simulink model "Sim_main"  (R2025a)
settings: Solver=FixedStepAuto  StartTime=0.0  StopTime=8760  FixedStep=1  RelTol=1e-3
values from neighbouring files (symbols this model uses):
  A = R * 2 * H    [LCOW_calculation.m]    (also in RUN_Simulink_POOL.m; RUN_Simulink_RandomSet.m; RUN_Simulink_SINGLE.m = 12.786871552)
  Cf = 36000    [RUN_Simulink_POOL.m]    (also in RUN_Simulink_RandomSet.m; RUN_Simulink_SINGLE.m)
  CutIn = 3    [RUN_Simulink_POOL.m]    (also in RUN_Simulink_RandomSet.m; RUN_Simulink_SINGLE.m)
  IP1 = (n/(n-1))*P1*( (P2/P1)^((n-1)/n) - 1)    (= 259255.992944)    [RUN_Simulink_POOL.m]    (also in RUN_Simulink_RandomSet.m; RUN_Simulink_SINGLE.m)
  J1 = 1.5 * As    [RUN_Simulink_POOL.m]    (also in RUN_Simulink_RandomSet.m; RUN_Simulink_SINGLE.m = 4.38)
  Limit_Tor = Tor_rq * 0.5    (= 2.3371585434)    [RUN_Simulink_POOL.m]    (also in RUN_Simulink_RandomSet.m; RUN_Simulink_SINGLE.m = 3.45899464424)
  N_PV = data.N_PV(i)    [LCOW_calculation.m]    (also in MOO_Qp_LCOW_CO2.m = optimvar("N_PV","Type","integer","LowerBound",1,"UpperBound"; RUN_Simulink_POOL.m = N_PV_values(i); RUN_Simulink_RandomSet.m = N_PV_values; RUN_Simulink_SINGLE.m = 2)
  N_ro = data.N_ro(i)    [LCOW_calculation.m]    (also in MOO_Qp_LCOW_CO2.m = optimvar("N_ro","Type","integer","LowerBound",2,"UpperBound"; RUN_Simulink_POOL.m = N_ro_values(i); RUN_Simulink_RandomSet.m = N_ro_values; RUN_Simulink_SINGLE.m = 6)
  Nt = data.Nt(i)    [LCOW_calculation.m]    (also in MOO_Qp_LCOW_CO2.m = optimvar("Nt","Type","integer","LowerBound",10,"UpperBound",; RUN_Simulink_POOL.m = Nt_values(i); RUN_Simulink_RandomSet.m = Nt_values; RUN_Simulink_SINGLE.m = 58)
  P2 = 800000    [RUN_Simulink_POOL.m]    (also in RUN_Simulink_RandomSet.m; RUN_Simulink_SINGLE.m)
  R = 0.515 * As    [LCOW_calculation.m]    (also in RUN_Simulink_POOL.m; RUN_Simulink_RandomSet.m; RUN_Simulink_SINGLE.m = 1.5038)
  Tor_rq = IP1 * Va * 10 / (17 * pi)    (= 4.67431708681)    [RUN_Simulink_POOL.m]    (also in RUN_Simulink_RandomSet.m; RUN_Simulink_SINGLE.m = 6.91798928848)
  TR = data.TR(i)    [LCOW_calculation.m]    (also in MOO_Qp_LCOW_CO2.m = optimvar("TR","LowerBound",3,"UpperBound",10); RUN_Simulink_POOL.m = TR_values(i); RUN_Simulink_RandomSet.m = TR_values; RUN_Simulink_SINGLE.m = 9.36)
  Va = e_vol * Vs    (= 9.6291546017e-05)    [RUN_Simulink_POOL.m]    (also in RUN_Simulink_RandomSet.m; RUN_Simulink_SINGLE.m = 0.000142511488105)
  Vf1 = ((P1+Pa)*T2/(T1*(P2+Pa)))*1000    (= 339.891157105)    [RUN_Simulink_POOL.m]    (also in RUN_Simulink_RandomSet.m; RUN_Simulink_SINGLE.m)
  Vt = 2000    [RUN_Simulink_POOL.m]    (also in RUN_Simulink_RandomSet.m; RUN_Simulink_SINGLE.m)
undefined symbols (not defined in the file or in its folder): magnitude
libraries: statsLibrary x36, simulink x1
(part 1 of 4)
settings Model: Creator=mep20kma  LastModifiedBy=mep20kma
settings DebuggingCC: AlgebraicLoopMsg=none

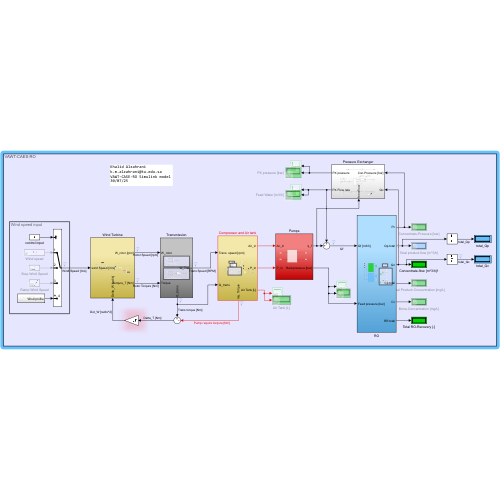
[thumbnail: Simulink's stored preview of the top-level diagram]
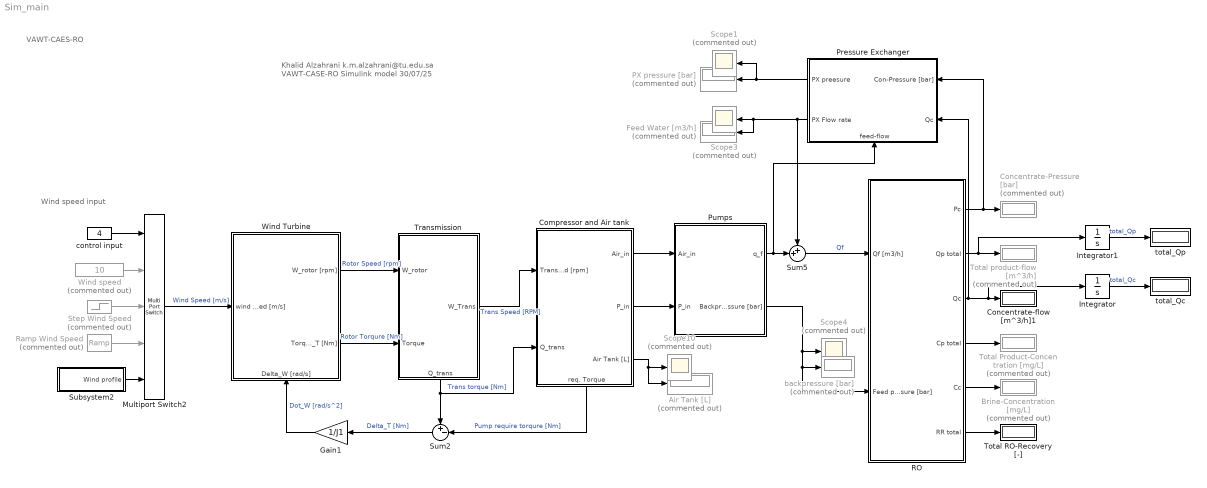
== system Sim_main ==
  note: Wind speed input
  note: VAWT-CAES-RO
  note: Khalid Alzahrani
      | k.m.alzahrani@tu.edu.sa
      | VAWT-CASE-RO Simulink model
      | 30/07/25
  Air Tank [L] : Display  Commented=on
      settings: Format=bank
  Brine-Concentration [mg/L] : Display  Commented=on
      settings: Format=bank
  Compressor and Air tank : Subsystem
      settings: PortSchema="{\"entries\":[{\"content\":{\"sides\":[{\"content\":{\"connectorIds\":[\"In1\",\"In2\"]},\"type\":\"ConnectorPlacement.EquallySpacedRectSide\",\"uuid\":\"bae99c5a-2a4b-4178-96fc-c8e23db237a2\"},{\"content\":{\"connectorIds\":[\"Out1\",\"Out2\",\"Out3\"],\"side\":\"RIGHT\"},\"type\":\"ConnectorPlacement.EquallySpacedRectSide\",\"uuid\":\"1992d0ba-6a8c-4d02-a787-c6c0cea2193f\"},{\"content\":{\"side\":\"TOP\"},\"type\":\"ConnectorPlacement.EquallySpacedRectSide\",\"uuid\":\"ca7b5cc6-18c4-4b8c-a524-0fed0e771665\"},{\"content\":{\"connectorIds\":[\"Out4\"],\"side\":\"BOTTOM\"},\"type\":\"ConnectorPlacement.EquallySpacedRectSide\",\"uuid\":\"cdfbee2c-ce1d-4f5d-a549-a4d701a0a4dd\"}]},\"type\":\"ConnectorPlacement.EquallySpacedConnector\",\"uuid\":\"eb75531c-d058-4587-8526-49bf71b34705\"}],\"packageUris\":[\"http://schema.mathworks.com/mf0/Connector/R2020b\"],\"version\":\"1.0\"}"
  Concentrate-Pressure [bar] : Display  Commented=on
  Concentrate-flow [m^3/h]1 : Display
      settings: Decimation=5
  Feed Water [m3/h] : Display  Commented=on
  Gain1 : Gain  Gain=1/J1
  Integrator : Integrator
  Integrator1 : Integrator  WrappedStateLowerValue=0.00000001
  Multiport Switch2 : MultiPortSwitch  Inputs=4  SaturateOnIntegerOverflow=off  InputSameDT=off
  PX pressure [bar] : Display  Commented=on
  Pressure Exchanger : Subsystem
      settings: PortSchema="{\"entries\":[{\"content\":{\"sides\":[{\"content\":{\"connectorIds\":[\"In1\",\"In2\"]},\"type\":\"ConnectorPlacement.EquallySpacedRectSide\",\"uuid\":\"0703a325-1e41-4562-9fad-9b159d1bd3be\"},{\"content\":{\"connectorIds\":[\"Out1\",\"Out2\"],\"side\":\"RIGHT\"},\"type\":\"ConnectorPlacement.EquallySpacedRectSide\",\"uuid\":\"c9b3212b-5369-47ef-bfa4-c3d90c4a3111\"},{\"content\":{\"side\":\"TOP\"},\"type\":\"ConnectorPlacement.EquallySpacedRectSide\",\"uuid\":\"f46ca4f0-02ad-4144-bb6a-e2761afa5cc2\"},{\"content\":{\"connectorIds\":[\"In3\"],\"side\":\"BOTTOM\"},\"type\":\"ConnectorPlacement.EquallySpacedRectSide\",\"uuid\":\"8b21c39f-2c5b-40be-94c0-35b7ce64feea\"}]},\"type\":\"ConnectorPlacement.EquallySpacedConnector\",\"uuid\":\"0ccfaa06-0329-44cf-a82f-b9aa7c53a6a3\"}],\"packageUris\":[\"http://schema.mathworks.com/mf0/Connector/R2020b\"],\"version\":\"1.0\"}"
  Pumps : Subsystem
  RO : Subsystem
  Ramp Wind Speed : simulink/Sources/Ramp  Commented=on  slope=0.1  start=0  InitialOutput=0
  Scope{1,3..4,10} (4 alike) : Scope  Commented=on
      Scope1 settings: ActiveDisplayYMinimum=-0.26427  ActiveDisplayYMaximum=2.37839  DataLoggingVariableName=ScopeData19
      Scope10 settings: ActiveDisplayYMinimum=-1627.2921760391182  ActiveDisplayYMaximum=23795.4869600652  DataLoggingVariableName=ScopeData22
      Scope3 settings: ActiveDisplayYMinimum=-6.500066936368408  ActiveDisplayYMaximum=58.500602427315691  DataLoggingVariableName=ScopeData32
      Scope4 settings: ActiveDisplayYMinimum=40.740007263636365  ActiveDisplayYMaximum=60.740007263636365  DataLoggingVariableName=ScopeData34
  Step Wind Speed : Step  Commented=on  After=6  SampleTime=1
  Subsystem2 : Subsystem
  Sum2 : Sum  Inputs=+-|
  Sum5 : Sum  Inputs=++|
  Total Product-Concentration [mg/L] : Display  Commented=on
  Total RO-Recovery [-] : Display
  Total product-flow [m^3/h] : Display  Commented=on
  Transmission : Subsystem
      settings: PortSchema="{\"entries\":[{\"content\":{\"sides\":[{\"content\":{\"connectorIds\":[\"In1\",\"In2\"]},\"type\":\"ConnectorPlacement.EquallySpacedRectSide\",\"uuid\":\"fe7cb8fe-c3d1-4fc2-abbc-e62d8a30f932\"},{\"content\":{\"connectorIds\":[\"Out1\"],\"side\":\"RIGHT\"},\"type\":\"ConnectorPlacement.EquallySpacedRectSide\",\"uuid\":\"d080c485-0a77-4f06-83bb-92ab059c673f\"},{\"content\":{\"connectorIds\":[],\"side\":\"TOP\"},\"type\":\"ConnectorPlacement.EquallySpacedRectSide\",\"uuid\":\"e27e7f1f-9635-4311-9c7d-d878089382ac\"},{\"content\":{\"connectorIds\":[\"Out2\"],\"side\":\"BOTTOM\"},\"type\":\"ConnectorPlacement.EquallySpacedRectSide\",\"uuid\":\"8768de16-74c5-42d8-8067-9fe7fba08fec\"}]},\"type\":\"ConnectorPlacement.EquallySpacedConnector\",\"uuid\":\"5aaf8406-eb77-4812-8f16-9b7078958fda\"}],\"packageUris\":[\"http://schema.mathworks.com/mf0/Connector/R2020b\"],\"version\":\"1.0\"}"
  Wind Turbine : Subsystem
      settings: PortSchema="{\"entries\":[{\"content\":{\"sides\":[{\"content\":{\"connectorIds\":[\"In1\"]},\"type\":\"ConnectorPlacement.EquallySpacedRectSide\",\"uuid\":\"fe7cb8fe-c3d1-4fc2-abbc-e62d8a30f932\"},{\"content\":{\"connectorIds\":[\"Out1\",\"Out2\"],\"side\":\"RIGHT\"},\"type\":\"ConnectorPlacement.EquallySpacedRectSide\",\"uuid\":\"d080c485-0a77-4f06-83bb-92ab059c673f\"},{\"content\":{\"connectorIds\":[],\"side\":\"TOP\"},\"type\":\"ConnectorPlacement.EquallySpacedRectSide\",\"uuid\":\"e27e7f1f-9635-4311-9c7d-d878089382ac\"},{\"content\":{\"connectorIds\":[\"In2\"],\"side\":\"BOTTOM\"},\"type\":\"ConnectorPlacement.EquallySpacedRectSide\",\"uuid\":\"c619a898-2bb3-4a9a-8369-a12a64617c75\"}]},\"type\":\"ConnectorPlacement.EquallySpacedConnector\",\"uuid\":\"5aaf8406-eb77-4812-8f16-9b7078958fda\"}],\"packageUris\":[\"http://schema.mathworks.com/mf0/Connector/R2020b\"],\"version\":\"1.0\"}"
  Wind speed : Constant  Commented=on  Value=10
  backpressure [bar] : Display  Commented=on
  control input : Constant  Value=4
  total_Qc : Display
      settings: Format=bank
  total_Qp : Display
      settings: Format=bank
  wires:
  Pressure Exchanger/2(PX Flow rate) -> Sum5/1, Feed Water [m3/h]/1, Scope3/1
  Compressor and Air tank/1(Air_in) -> Pumps/1(Air_in)
  Sum2/1 -> Gain1/1  "Delta_T [Nm]"
  Sum5/1 -> RO/1(Qf [m3/h])  "Qf"
  RO/2(Qp total) -> Integrator1/1, Total product-flow [m^3/h]/1
  Pumps/2(Backpressure [bar]) -> RO/2(Feed pressure [bar]), backpressure [bar]/1, Scope4/1
  Multiport Switch2/1 -> Wind Turbine/1(wind Speed [m/s])  "Wind Speed [m/s]"
  Compressor and Air tank/3(Air Tank [L]) -> Air Tank [L]/1, Scope10/1
  Transmission/1(W_Trans) -> Compressor and Air tank/1(Trans. speed [rpm])  "Trans Speed [RPM]"
  Compressor and Air tank/4(req. Torque) -> Sum2/2  "Pump require torqure [Nm]"
  Pressure Exchanger/1(PX preesure) -> Scope1/1, PX pressure [bar]/1
  Integrator1/1 -> total_Qp/1  "total_Qp"
  RO/5(Cc) -> Brine-Concentration [mg/L]/1
  Transmission/2(Q_trans) -> Compressor and Air tank/2(Q_trans), Sum2/1  "Trans torque [Nm]"
  Ramp Wind Speed/1 -> Multiport Switch2/4
  RO/3(Qc) -> Integrator/1, Concentrate-flow [m^3/h]1/1, Pressure Exchanger/2(Qc)
  RO/1(Pc) -> Concentrate-Pressure [bar]/1, Pressure Exchanger/1(Con-Pressure [bar])
  Wind speed/1 -> Multiport Switch2/2
  Wind Turbine/2(Torqure_T [Nm]) -> Transmission/2(Torque)  "Rotor Torqure [Nm]"
  Subsystem2/1(Wind profile) -> Multiport Switch2/5
  Wind Turbine/1(W_rotor [rpm]) -> Transmission/1(W_rotor)  "Rotor Speed [rpm]"
  Gain1/1 -> Wind Turbine/2(Delta_W [rad/s])  "Dot_W [rad/s^2]"
  Compressor and Air tank/2(P_in) -> Pumps/2(P_in)
  control input/1 -> Multiport Switch2/1
  RO/4(Cp total) -> Total Product-Concentration [mg/L]/1
  RO/6(RR total) -> Total RO-Recovery [-]/1
  Step Wind Speed/1 -> Multiport Switch2/3
  Pumps/1(q_f) -> Sum5/2, Pressure Exchanger/3(feed-flow)
  Integrator/1 -> total_Qc/1  "total_Qc"

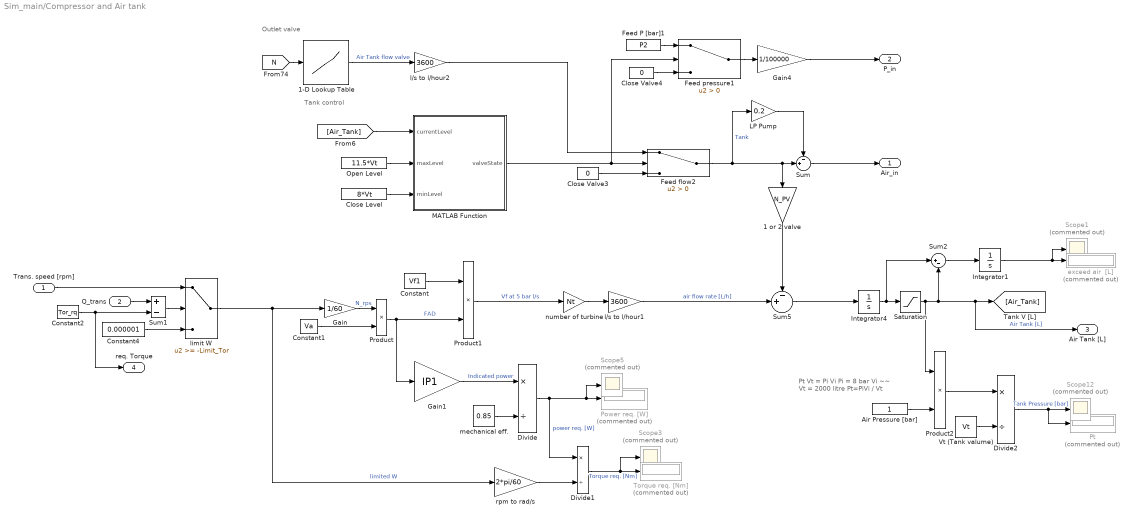
== system Sim_main/Compressor and Air tank ==
  note: Tank control
  note: Outlet valve
  note: Pt Vt = Pi Vi
      | Pi = 8 bar
      | Vi ~~
      | Vt = 2000 litre
      |
      | Pt=PiVi / Vt
  Trans. speed [rpm] : Inport
  Q_trans : Inport  Port=2
  1 or 2 valve : Gain  Gain=N_PV
  1-D Lookup Table : Lookup_n-D  NumberOfTableDimensions=1  BreakpointsForDimension1=[1;2;3;4;5;6]  Table=[9.33;11.38;12.28;12.77;13.07;13.25]  InternalRulePriority=Speed  RndMeth=Simplest
  Air Pressure [bar] : Constant
  Close Level : Constant  Value=8*Vt
  Close Valve3 : Constant  Value=0
  Close Valve4 : Constant  Value=0
  Constant : Constant  Value=Vf1
  Constant1 : Constant  Value=Va
  Constant2 : Constant  Value=Tor_rq
  Constant4 : Constant  Value=0.000001
  Divide : Product  Inputs=*/
  Divide1 : Product  Inputs=*/
  Divide2 : Product  Inputs=*/
  Feed P [bar]1 : Constant  Value=P2
  Feed flow2 : Switch  Criteria=u2 > Threshold  ZeroCross=off  SaturateOnIntegerOverflow=off  InputSameDT=off
  Feed pressure1 : Switch  Criteria=u2 > Threshold  ZeroCross=off  SaturateOnIntegerOverflow=off  InputSameDT=off
  Gain : Gain  Gain=1/60
  Gain1 : Gain  Gain=IP1
  Gain4 : Gain  Gain=1/100000
  Integrator1 : Integrator  LimitOutput=on  LowerSaturationLimit=0
  Integrator4 : Integrator  UpperSaturationLimit=2000  LowerSaturationLimit=0
  LP Pump : Gain  Gain=0.2
  MATLAB Function : MATLAB Function  TreatAsAtomicUnit=on
  Open Level : Constant  Value=11.5*Vt
  Power req. [W] : Display  Commented=on
  Product : Product
  Product1 : Product
  Product2 : Product
  Pt : Display  Commented=on
  Saturation : Saturate  UpperLimit=11.5*Vt  LowerLimit=0
  Scope{1,3,5,12} (4 alike) : Scope  Commented=on
      Scope1 settings: ActiveDisplayYMinimum=-793541.28733564925  ActiveDisplayYMaximum=88171.254148405453  DataLoggingVariableName=ScopeData43
      Scope12 settings: ActiveDisplayYMinimum=-1.4374999999999998  ActiveDisplayYMaximum=12.9375
      Scope3 settings: ActiveDisplayYMinimum=4.674317086807517  ActiveDisplayYMaximum=4.67431708680752  DataLoggingVariableName=ScopeData3
      Scope5 settings: ActiveDisplayYMinimum=0.912  ActiveDisplayYMaximum=2.912  DataLoggingVariableName=ScopeData2
  Sum : Sum  Inputs=-+|
  Sum1 : Sum  Inputs=+-
  Sum2 : Sum  Inputs=|+-
  Sum5 : Sum  Inputs=-+|
  Torque req. [Nm] : Display  Commented=on
  Vt (Tank valume) : Constant  Value=Vt
  exceed air  [L] : Display  Commented=on
      settings: Format=bank
  l/s to l/hour1 : Gain  Gain=3600
  l/s to l/hour2 : Gain  Gain=3600
  limit W : Switch  Threshold=-Limit_Tor  SaturateOnIntegerOverflow=off  InputSameDT=off
  mechanical eff. : Constant  Value=0.85
  number of turbine : Gain  Gain=Nt
  rpm to rad/s : Gain  Gain=2*pi/60
  Air_in : Outport
  P_in : Outport  Port=2
  Air Tank [L] : Outport  Port=3
  req. Torque : Outport  Port=4
  wires:
  Saturation/1 -> [Air_Tank], Air Tank [L]/1, Sum2/2, Product2/1  "Air Tank [L]"
  Integrator4/1 -> Saturation/1, Sum2/1
  LP Pump/1 -> Sum/1
  Sum/1 -> Air_in/1
  number of turbine/1 -> l/s to l/hour1/1
  Product1/1 -> number of turbine/1  "Vf at 5 bar l/s"
  Constant1/1 -> Product/2
  Divide/1 -> Scope5/1, Power req. [W]/1, Divide1/1  "power req. [W]"
  Gain1/1 -> Divide/1  "Indicated power"
  mechanical eff./1 -> Divide/2
  Divide1/1 -> Scope3/1, Torque req. [Nm]/1  "Torque req. [Nm]"
  rpm to rad/s/1 -> Divide1/2
  Gain/1 -> Product/1  "N_rps"
  Product/1 -> Gain1/1, Product1/2  "FAD"
  Constant/1 -> Product1/1
  Sum5/1 -> Integrator4/1
  l/s to l/hour1/1 -> Sum5/2  "air flow rate [L/h]"
  Gain4/1 -> P_in/1
  1-D Lookup Table/1 -> l/s to l/hour2/1  "Air Tank flow valve"
  Close Valve3/1 -> Feed flow2/3
  Feed flow2/1 -> Sum/2, 1 or 2 valve/1, LP Pump/1  "Tank"
  Feed pressure1/1 -> Gain4/1
  Close Valve4/1 -> Feed pressure1/3
  Feed P [bar]1/1 -> Feed pressure1/1
  [Air_Tank] -> MATLAB Function/1(currentLevel)
  Open Level/1 -> MATLAB Function/2(maxLevel)
  Close Level/1 -> MATLAB Function/3(minLevel)
  limit W/1 -> Gain/1, rpm to rad/s/1  "limited W"
  Air Pressure [bar]/1 -> Product2/2
  Product2/1 -> Divide2/1
  Vt (Tank valume)/1 -> Divide2/2
  Divide2/1 -> Pt/1, Scope12/1  "Tank Pressure [bar]"
  [N] -> 1-D Lookup Table/1
  MATLAB Function/1(valveState) -> Feed pressure1/2, Feed flow2/2
  Constant4/1 -> limit W/3
  Trans. speed [rpm]/1 -> limit W/1
  Constant2/1 -> Sum1/2, req. Torque/1
  Q_trans/1 -> Sum1/1
  Sum2/1 -> Integrator1/1
  Integrator1/1 -> Scope1/1, exceed air  [L]/1
  l/s to l/hour2/1 -> Feed flow2/1
  1 or 2 valve/1 -> Sum5/1
  Sum1/1 -> limit W/2

== system Sim_main/Pressure Exchanger ==
  Con-Pressure [bar] : Inport
  Qc : Inport  Port=2
  feed-flow : Inport  Port=3
  1-D Lookup Table : Lookup_n-D  NumberOfTableDimensions=1  BreakpointsForDimension1=[2.07;2.68;2.988;3.148;3.242;3.299]  Table=[10.87;8.244;7.039;6.335;5.916;5.636]  InternalRulePriority=Speed  RndMeth=Simplest
  Constant3 : Constant  Value=0
  Display{1..2,9..11} (5 alike) : Display
      Display2 settings: Format=bank
  Memory : Memory  InitialCondition=10
  Saturation : Saturate  UpperLimit=inf  LowerLimit=0
  Scope1 : Scope  Commented=on
      settings: ActiveDisplayYMinimum=-11.877690131011091  ActiveDisplayYMaximum=106.89921117909984  DataLoggingVariableName=ScopeData15
  Switch3 : Switch  Criteria=u2 > Threshold  SaturateOnIntegerOverflow=off  InputSameDT=off
  eff flow rate1 : Gain  Gain=0.96
  eff flow rate3 : Gain  Gain=0.96
  eff pressure : Gain  Gain=0.99
  PX preesure : Outport
  PX Flow rate : Outport  Port=2
  wires:
  Con-Pressure [bar]/1 -> eff pressure/1
  eff pressure/1 -> PX preesure/1
  1-D Lookup Table/1 -> Display9/1, Switch3/1
  eff flow rate1/1 -> PX Flow rate/1, Display11/1
  Constant3/1 -> Switch3/3
  Switch3/1 -> eff flow rate1/1
  Memory/1 -> eff flow rate3/1
  Qc/1 -> Scope1/1, Display2/1, Saturation/1
  feed-flow/1 -> 1-D Lookup Table/1, Display10/1, Switch3/2
  Saturation/1 -> Memory/1
  eff flow rate3/1 -> Display1/1

== system Sim_main/Pumps ==
  Air_in : Inport
  P_in : Inport  Port=2
  Air operated pump : Subsystem
  q_f : Outport
  Backpressure [bar] : Outport  Port=2
  wires:
  Air operated pump/1(Feed flow m3/h) -> q_f/1
  Air_in/1 -> Air operated pump/1(Air_in)
  Air operated pump/2(Backpressure [bar]) -> Backpressure [bar]/1
  P_in/1 -> Air operated pump/2(P_in)

== system Sim_main/RO ==
  note: Number of RO
  Qf [m3/h] : Inport
  Feed pressure [bar] : Inport  Port=2
  Add1 : Sum
  Add4 : Sum
  Constant : Constant  Value=N_PV
  Constant1 : Constant  Value=N_PV
  Constant2 : Constant  Value=N_ro
  Display{,1..5} (6 alike) : Display  Commented=on
      settings: Format=bank
  Display6 : Display
      settings: Format=bank
  Gain : Gain  Gain=2
  Integrator : Integrator
  PV1 : Subsystem
  PV2 : Subsystem
  Qp : MultiPortSwitch  Inputs=2  SaturateOnIntegerOverflow=off  InputSameDT=off
  Qp1 : MultiPortSwitch  Inputs=2  SaturateOnIntegerOverflow=off  InputSameDT=off
  Pc : Outport
  Qp total : Outport  Port=2
  Qc : Outport  Port=3
  Cp total : Outport  Port=4
  Cc : Outport  Port=5
  RR total : Outport  Port=6
  tag scope: N=global
  wires:
  Qf [m3/h]/1 -> PV1/1(Qf [m3/h]), PV2/1(Qf [m3/h]), Gain/1
  PV1/4(Cp total) -> Cp total/1
  Feed pressure [bar]/1 -> PV2/2(Feed pressure [bar]), PV1/2(Feed pressure [bar])
  PV1/1(Pc) -> Pc/1
  PV1/6(RR total) -> RR total/1  "total_RR"
  PV1/5(Cc) -> Cc/1
  PV1/3(Qc) -> [Qc1]
  Add4/1 -> Qp/3
  PV1/2(Qp total) -> [Qp1]
  PV2/2(Qp total) -> [Qp2]
  PV2/3(Qc) -> [Qc2]
  PV2/1(Pc) -> Display/1
  PV2/4(Cp total) -> Display1/1
  PV2/5(Cc) -> Display2/1
  PV2/6(RR total) -> Display3/1
  [Qp1] -> Add4/1
  [Qp2] -> Add4/2
  Add1/1 -> Qp1/3
  [Qc1] -> Add1/1
  [Qc2] -> Add1/2
  Constant/1 -> Qp/1
  [Qp1] -> Qp/2
  Qp/1 -> Qp total/1, Display4/1  "Qp"
  Qp1/1 -> Qc/1, Display5/1  "Qc"
  Constant1/1 -> Qp1/1
  [Qc1] -> Qp1/2
  Constant2/1 -> [N]
  Integrator/1 -> Display6/1  "total_Qf"
  Gain/1 -> Integrator/1
